simulink model "quad_sim_mult_UAVs_coop_localization"  (R2017a)
settings: Solver=VariableStepAuto  StartTime=0.0  StopTime=60  FixedStep=0.02  MaxStep=0.03  MinStep=0.02  RelTol=1e-3  EnableMultiTasking=on
InitFcn:
  | setup_gains
  | % --- Outer loop gains --------
  | %P_X=9.44;   I_X=0.23;  D_X=2.36;
  | %P_Y=9.33;   I_Y=0.18;  D_Y=1.54;
  | % --------------------------
  | 
  | %CARLA TUNNED PID
  | %P_Z = 51.037;       I_Z = 43.051;        D_Z = 11.771;
  | %P_Z = 0.5;       I_Z = 0.15;        D_Z = 0.2;
  | %P_Z = 32.55;       I_Z = 9.82;        D_Z = 4.65 ;
  | 
  | global clientID;
  | clientID=-1;
values from neighbouring files (symbols this model uses):
  End_POS_coop = Start_POS+0.5    [setup_gains.m]
  Kd_az = 0.001    [setup_gains.m]
  Kd_px = 0.5    [setup_gains.m]
  Kd_py = 0.5    [setup_gains.m]
  Kd_pz = 0.025    [setup_gains.m]
  Kd_vx = 2    [setup_gains.m]
  Kd_vy = 2    [setup_gains.m]
  Kd_vz = 0.05    [setup_gains.m]
  Ki_az = 0.01    [setup_gains.m]
  Ki_px = 0.001    [setup_gains.m]
  Ki_py = 0.001    [setup_gains.m]
  Ki_pz = 0.001    [setup_gains.m]
  Ki_vx = 0.1    [setup_gains.m]
  Ki_vy = 0.1    [setup_gains.m]
  Ki_vz = 2.5    [setup_gains.m]
  Kp_az = 0.75    [setup_gains.m]
  Kp_px = 1    [setup_gains.m]
  Kp_py = 1    [setup_gains.m]
  Kp_pz = 0.5    [setup_gains.m]
  Kp_vx = 15.00    (= 15)    [setup_gains.m]
  Kp_vy = 15.00    (= 15)    [setup_gains.m]
  Kp_vz = 5    [setup_gains.m]
  s1 = cputime()*10    [setup_gains.m]
  s2 = round(s1+randn*10 + 1)    [setup_gains.m]
  s3 = round(s2+randn*10 + 32)    [setup_gains.m]
  s4 = round(s3+randn*10 + 55)    [setup_gains.m]
  Start_POS = [ -1.00 -1.00 1.05 ... (first row only)    [setup_gains.m]
  var_accel = 0.0001    [setup_gains.m]
  var_pos = 0.5^2    (= 0.25)    [setup_gains.m]
  var_ranges = 0.0025    [setup_gains.m]
undefined symbols (not defined in the file or in its folder): W, X, Y, Z
libraries: dspindex x15, robotlib x13, dspsigops x12
(part 2 of 2)

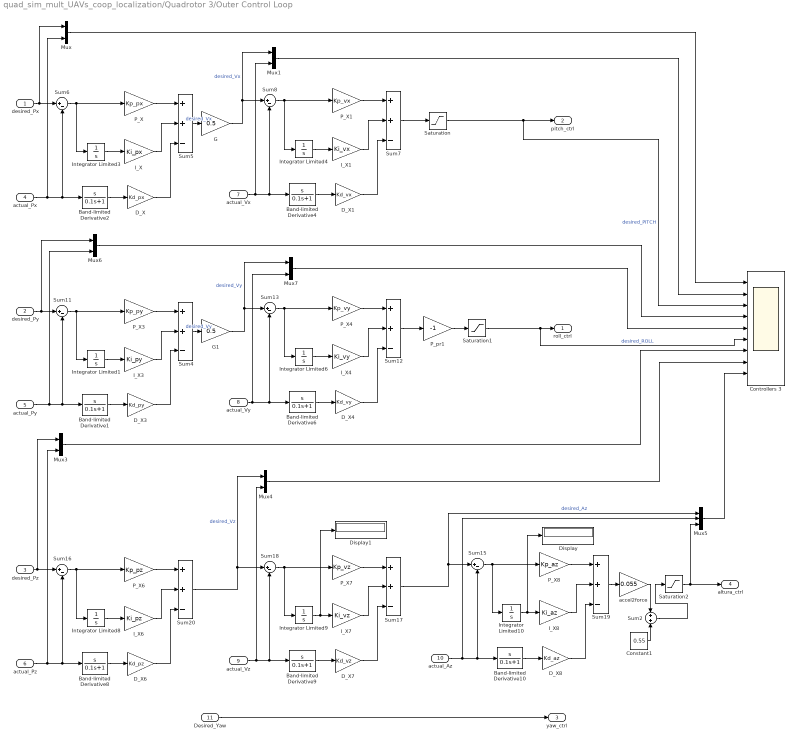
== system quad_sim_mult_UAVs_coop_localization/Quadrotor 3/Outer Control Loop ==
  desired_Px : Inport
  desired_Py : Inport  Port=2
  desired_Pz : Inport  Port=3
  actual_Px : Inport  Port=4
  actual_Py : Inport  Port=5
  actual_Pz : Inport  Port=6
  actual_Vx : Inport  Port=7
  actual_Vy : Inport  Port=8
  actual_Vz : Inport  Port=9
  actual_Az : Inport  Port=10
  Desired_Yaw : Inport  Port=11
  Band-limited Derivative{1..2,4,6,8..10} (7 alike) : TransferFcn  Numerator=[1 0]  Denominator=[0.1 1]
  Constant1 : Constant  Value=0.55
  Controllers 3 : Scope  NumInputPorts=9
  D_X : Gain  Gain=Kd_px
  D_X1 : Gain  Gain=Kd_vx
  D_X3 : Gain  Gain=Kd_py
  D_X4 : Gain  Gain=Kd_vy
  D_X6 : Gain  Gain=Kd_pz
  D_X7 : Gain  Gain=Kd_vz
  D_X8 : Gain  Gain=Kd_az
  Display : Display
  Display1 : Display
  G : Gain  Gain=0.5
  G1 : Gain  Gain=0.5
  I_X : Gain  Gain=Ki_px
  I_X1 : Gain  Gain=Ki_vx
  I_X3 : Gain  Gain=Ki_py
  I_X4 : Gain  Gain=Ki_vy
  I_X6 : Gain  Gain=Ki_pz
  I_X7 : Gain  Gain=Ki_vz
  I_X8 : Gain  Gain=Ki_az
  Integrator Limited{1,3..4,6} (4 alike) : Integrator  LimitOutput=on  UpperSaturationLimit=100  LowerSaturationLimit=-100
  Integrator Limited10 : Integrator  LimitOutput=on  UpperSaturationLimit=1000  LowerSaturationLimit=-1000
  Integrator Limited8 : Integrator  LimitOutput=on  UpperSaturationLimit=1000  LowerSaturationLimit=-1000
  Integrator Limited9 : Integrator  LimitOutput=on  UpperSaturationLimit=1000  LowerSaturationLimit=-1000
  Mux{,1,3..4,6..7} (6 alike) : Mux  Inputs=2
  Mux5 : Mux  Inputs=3
  P_X : Gain  Gain=Kp_px
  P_X1 : Gain  Gain=Kp_vx
  P_X3 : Gain  Gain=Kp_py
  P_X4 : Gain  Gain=Kp_vy
  P_X6 : Gain  Gain=Kp_pz
  P_X7 : Gain  Gain=Kp_vz
  P_X8 : Gain  Gain=Kp_az
  P_pr1 : Gain  Gain=-1
  Saturation : Saturate  UpperLimit=2  LowerLimit=-2
  Saturation1 : Saturate  UpperLimit=2  LowerLimit=-2
  Saturation2 : Saturate  UpperLimit=10  LowerLimit=0
  Sum{6,8,11,13,15..16,18} (7 alike) : Sum  Inputs=|+-
  Sum{4..5,7,12,17,19..20} (7 alike) : Sum  Inputs=++-
  Sum2 : Sum  Inputs=+|+
  accel2force : Gain  Gain=0.055
  roll_ctrl : Outport
  pitch_ctrl : Outport  Port=2
  yaw_ctrl : Outport  Port=3
  altura_ctrl : Outport  Port=4
  wires:
  Saturation1/1 -> Controllers 3/6, roll_ctrl/1  "desired_ROLL"
  Saturation/1 -> Controllers 3/3, pitch_ctrl/1  "desired_PITCH"
  P_pr1/1 -> Saturation1/1
  Mux7/1 -> Controllers 3/5
  Mux6/1 -> Controllers 3/4
  actual_Vy/1 -> Mux7/2, Sum13/2, Band-limited Derivative6/1
  desired_Py/1 -> Sum11/1, Mux6/1
  actual_Py/1 -> Mux6/2, Band-limited Derivative1/1, Sum11/2
  Constant1/1 -> Sum2/2
  accel2force/1 -> Sum2/1
  Sum2/1 -> Saturation2/1
  Sum19/1 -> accel2force/1
  Mux5/1 -> Controllers 3/9
  Mux4/1 -> Controllers 3/8
  Mux3/1 -> Controllers 3/7
  Sum17/1 -> Sum15/1, Mux5/1  "desired_Az"
  actual_Az/1 -> Sum15/2, Band-limited Derivative10/1, Mux5/2
  Sum20/1 -> Sum18/1, Mux4/1  "desired_Vz"
  actual_Vz/1 -> Band-limited Derivative9/1, Sum18/2, Mux4/2
  Mux1/1 -> Controllers 3/2
  Mux/1 -> Controllers 3/1
  I_X8/1 -> Sum19/2
  Band-limited Derivative10/1 -> D_X8/1
  D_X8/1 -> Sum19/3
  P_X8/1 -> Sum19/1
  Integrator Limited10/1 -> I_X8/1, Display/1
  Sum15/1 -> P_X8/1, Integrator Limited10/1
  I_X7/1 -> Sum17/2
  Band-limited Derivative9/1 -> D_X7/1
  D_X7/1 -> Sum17/3
  P_X7/1 -> Sum17/1
  Integrator Limited9/1 -> I_X7/1, Display1/1
  Sum18/1 -> Integrator Limited9/1, P_X7/1
  I_X6/1 -> Sum20/2
  desired_Pz/1 -> Sum16/1, Mux3/1
  Band-limited Derivative8/1 -> D_X6/1
  actual_Pz/1 -> Sum16/2, Band-limited Derivative8/1, Mux3/2
  D_X6/1 -> Sum20/3
  P_X6/1 -> Sum20/1
  Integrator Limited8/1 -> I_X6/1
  Sum16/1 -> P_X6/1, Integrator Limited8/1
  Sum12/1 -> P_pr1/1
  G1/1 -> Mux7/1, Sum13/1  "desired_Vy"
  I_X4/1 -> Sum12/2
  Band-limited Derivative6/1 -> D_X4/1
  D_X4/1 -> Sum12/3
  P_X4/1 -> Sum12/1
  Integrator Limited6/1 -> I_X4/1
  Sum13/1 -> P_X4/1, Integrator Limited6/1
  I_X3/1 -> Sum4/2
  Band-limited Derivative1/1 -> D_X3/1
  D_X3/1 -> Sum4/3
  P_X3/1 -> Sum4/1
  Integrator Limited1/1 -> I_X3/1
  Sum11/1 -> Integrator Limited1/1, P_X3/1
  Sum7/1 -> Saturation/1
  G/1 -> Sum8/1, Mux1/1  "desired_Vx"
  I_X1/1 -> Sum7/2
  Band-limited Derivative4/1 -> D_X1/1
  actual_Vx/1 -> Band-limited Derivative4/1, Sum8/2, Mux1/2
  D_X1/1 -> Sum7/3
  P_X1/1 -> Sum7/1
  Integrator Limited4/1 -> I_X1/1
  Sum8/1 -> Integrator Limited4/1, P_X1/1
  Saturation2/1 -> altura_ctrl/1, Mux5/3
  I_X/1 -> Sum5/2
  desired_Px/1 -> Sum6/1, Mux/1
  Band-limited Derivative2/1 -> D_X/1
  actual_Px/1 -> Sum6/2, Band-limited Derivative2/1, Mux/2
  D_X/1 -> Sum5/3
  P_X/1 -> Sum5/1
  Integrator Limited3/1 -> I_X/1
  Sum6/1 -> P_X/1, Integrator Limited3/1
  Desired_Yaw/1 -> yaw_ctrl/1
  Sum5/1 -> G/1  "desired_Vx"
  Sum4/1 -> G1/1  "desired_Vy"

== system quad_sim_mult_UAVs_coop_localization/Quadrotor 3/Quadrirrotor Communication ==
  roll : Inport
  pitch : Inport  Port=2
  yaw : Inport  Port=3
  throttle : Inport  Port=4
  Blank Message : robotlib/Blank Message  SourceLibraryInfo=This block requires Robotics System Toolbox  messageType=geometry_msgs/Quaternion  SampleTime=inf
      settings: SourceProductBaseCode=RO
  Bus Assignment1 : BusAssignment  DialogController=Simulink.DDGSource_BusAssignment  AssignedSignals=X,Y,Z,W
  Bus Selector1 : BusSelector  OutputSignals=Data
  Data Type Conversion : DataTypeConversion  OutDataTypeStr=double
  Multiport Selector : dspindex/Multiport Selector  rowsOrCols=Rows  idxCellArray={ 1,2,3,4,5,6,7,8,9}  idxErrMode=Generate Error
  Publish2 : robotlib/Publish  SourceLibraryInfo=This block requires Robotics System Toolbox  topicSource=Specify your own  topic=/commands_attitude_3  messageType=geometry_msgs/Quaternion  messageQueueLength=105
      settings: SourceProductBaseCode=RO
  Subscribe : robotlib/Subscribe  SourceLibraryInfo=This block requires Robotics System Toolbox  topicSource=Specify your own  topic=/quadrotor_states_3  messageType=std_msgs/Float32MultiArray  sampleTime=-1  messageQueueLength=51
      settings: SourceProductBaseCode=RO
  Terminator : Terminator
  quad_pos_x : Outport
  quad_pos_y : Outport  Port=2
  quad_pos_z : Outport  Port=3
  quad_vel_x : Outport  Port=4
  quad_vel_y : Outport  Port=5
  quad_vel_z : Outport  Port=6
  quad_acc_x : Outport  Port=7
  quad_acc_y : Outport  Port=8
  quad_acc_z : Outport  Port=9
  wires:
  roll/1 -> Bus Assignment1/2
  pitch/1 -> Bus Assignment1/3
  yaw/1 -> Bus Assignment1/4
  throttle/1 -> Bus Assignment1/5
  Bus Selector1/1 -> Data Type Conversion/1  "<Data>"
  Data Type Conversion/1 -> Multiport Selector/1
  Multiport Selector/6 -> quad_vel_z/1
  Multiport Selector/5 -> quad_vel_y/1
  Multiport Selector/4 -> quad_vel_x/1
  Multiport Selector/3 -> quad_pos_z/1
  Multiport Selector/2 -> quad_pos_y/1
  Multiport Selector/1 -> quad_pos_x/1
  Bus Assignment1/1 -> Publish2/1
  Subscribe/2 -> Bus Selector1/1
  Subscribe/1 -> Terminator/1
  Blank Message/1 -> Bus Assignment1/1
  Multiport Selector/7 -> quad_acc_x/1
  Multiport Selector/8 -> quad_acc_y/1
  Multiport Selector/9 -> quad_acc_z/1
